simulink model "step_test2"  (Simulink 7.9)
settings: Solver=ode3  StartTime=0.0  StopTime=40  FixedStep=0.001  RelTol=1e-3
values from neighbouring files (symbols this model uses):
  den = [1 5.18 14.12]    [Project_Model_Params.m]    (also in Ziegler_Nichols_0.m = [0.05 1.7185 16.71 49.88 61.35 0]; step_test_params.m = [1 14.37 46.82 61.35])
  int_max = 150    [Project_Model_Params.m]    (also in step_test_params.m = 1000)
  int_min = -150    [Project_Model_Params.m]    (also in step_test_params.m = -1000)
  Kd = Kp*0.125*P_cr    (= 0.532770091731)    [Project_Model_Params.m]    (also in Ziegler_Nichols_0.m = 0.762550216826; step_test_params.m = 0.955086194687)
  Ki = Kp*2/P_cr    (= 2.12892018077)    [Project_Model_Params.m]    (also in Ziegler_Nichols_0.m = 4.58089306504; step_test_params.m = 3.46055049103)
  Kp = 0.6*K_cr    (= 2.13)    [Project_Model_Params.m]    (also in Ziegler_Nichols_0.m = 3.738; step_test_params.m = 3.636)
  num = [15.12]    [Project_Model_Params.m]    (also in Ziegler_Nichols_0.m = [-0.803 13.874 43.72]; step_test_params.m = [16.06 43.72])
  Ts = 0.1    [Project_Model_Params.m]    (also in step_test_params.m)
settings Model: Creator=gomi  LastModifiedBy=quchao

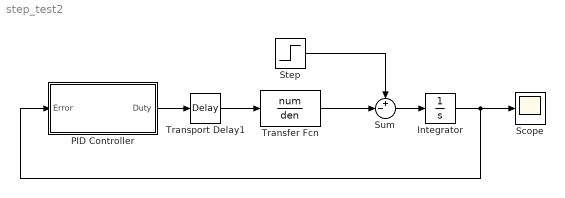
== system step_test2 ==
  Integrator : Integrator
  PID Controller : Subsystem
  Scope : Scope
  Step : Step  SampleTime=0
  Sum : Sum  Inputs=+-|
  Transfer Fcn : TransferFcn  Numerator=num  Denominator=den
  Transport Delay1 : TransportDelay  DelayTime=Ts
  wires:
  PID Controller/1(Duty) -> Transport Delay1/1
  Transport Delay1/1 -> Transfer Fcn/1
  Transfer Fcn/1 -> Sum/2
  Step/1 -> Sum/1
  Sum/1 -> Integrator/1
  Integrator/1 -> PID Controller/1(Error), Scope/1

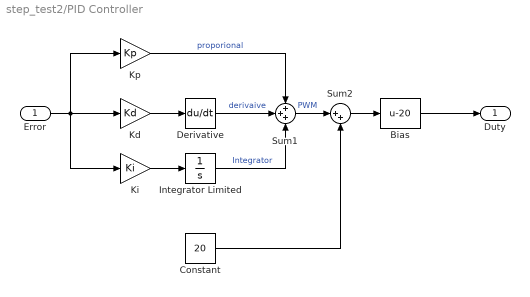
== system step_test2/PID Controller ==
  Error : Inport
  Bias : Bias  Bias=-20
  Constant : Constant  Value=20
  Derivative : Derivative
  Integrator Limited : Integrator  LimitOutput=on  UpperSaturationLimit=int_max  LowerSaturationLimit=int_min
  Kd : Gain  Gain=Kd
  Ki : Gain  Gain=Ki
  Kp : Gain  Gain=Kp
  Sum1 : Sum  Inputs=+++
  Sum2 : Sum  Inputs=|++
  Duty : Outport
  wires:
  Error/1 -> Kd/1, Kp/1, Ki/1
  Integrator Limited/1 -> Sum1/3  "Integrator"
  Derivative/1 -> Sum1/2  "derivaive"
  Kp/1 -> Sum1/1  "proporional"
  Ki/1 -> Integrator Limited/1
  Kd/1 -> Derivative/1
  Sum1/1 -> Sum2/1  "PWM"
  Sum2/1 -> Bias/1
  Constant/1 -> Sum2/2
  Bias/1 -> Duty/1
